simulink model "Simulink_Simulation"  (R2020a)
settings: Solver=ode23tb  StartTime=0.0  StopTime=10.0  RelTol=1e-3  EnableMultiTasking=on
undefined symbols (not defined in the file or in its folder): sigbuilder_block
libraries: powerlib x8
settings Model: Creator=LENOVO  LastModifiedBy=x64
settings DataIOCC: LimitDataPoints=on  SaveFormat=Array  ReturnWorkspaceOutputs=off
settings OptimizationCC: LifeSpan=inf
settings DebuggingCC: SolverPrmCheckMsg=warning  SFUnexpectedBacktrackingDiag=warning  SFNoUnconditionalDefaultTransitionDiag=warning  SFExecutionAtInitializationDiag=none  ArithmeticOperatorsInVariantConditions=warning
settings HardwareCC: ProdBitPerPointer=32  ProdBitPerSizeT=32  ProdBitPerPtrDiffT=32  ProdLargestAtomicFloat=None  ProdIntDivRoundTo=Undefined  ProdEndianess=Unspecified  ProdWordSize=32  ProdHWDeviceType=32-bit Generic
settings ModelReferenceCC: PropagateSignalLabelsOutOfModel=off
settings SFSimCC: SimUseLocalCustomCode=off  CustomCodeUndefinedFunction=UseInterfaceOnly
settings RTWCC: RTWUseLocalCustomCode=off
settings CodeAppCC: StateflowObjectComments=on
settings GRTTargetCC: TargetLangStandard=C89/C90 (ANSI)
settings ConfigComp: CovMetricSettings=dw  CovHtmlReporting=on  CovSaveCumulativeToWorkspaceVar=on  CovSaveSingleToWorkspaceVar=on  CovExternalEMLEnable=off  CovSFcnEnable=off
settings SimscapeCC: SimscapeNormalizeSystem=off

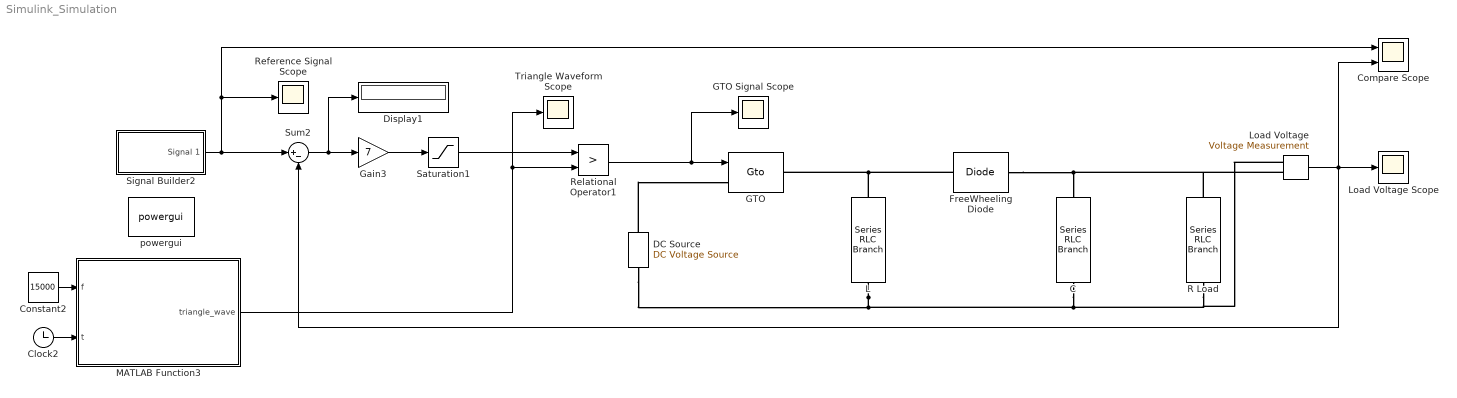
== system Simulink_Simulation ==
  " L" : powerlib/Elements/Series RLC Branch  LConnTagsString=__new0  RConnTagsString=__new0  BranchType=L  Resistance=1  Inductance=3*(1e-4)  SetiL0=off  InitialCurrent=0  Capacitance=1e-6  Setx0=off  InitialVoltage=0  Measurements=None
  " R Load" : powerlib/Elements/Series RLC Branch  LConnTagsString=__new0  RConnTagsString=__new0  BranchType=R  Resistance=100  Inductance=1e-3  SetiL0=off  InitialCurrent=0  Capacitance=1e-6  Setx0=off  InitialVoltage=0  Measurements=None
  C : powerlib/Elements/Series RLC Branch  LConnTagsString=__new0  RConnTagsString=__new0  BranchType=C  Resistance=1  Inductance=1e-3  SetiL0=off  InitialCurrent=0  Capacitance=(1e-6)*250  Setx0=off  InitialVoltage=0  Measurements=None
  Clock2 : Clock
  Compare Scope : Scope  NumInputPorts=2
  Constant2 : Constant  Value=15000
  DC Source : powerlib/Electrical Sources/DC Voltage Source  Amplitude=15  Measurements=None
  Display1 : Display
  FreeWheeling Diode : powerlib/Power Electronics/Diode  Ron=0.01  Lon=0.01  Vf=1  IC=0  UseSnubber=off  Rs=5000  Cs=250e-2  Measurements=off
  GTO : powerlib/Power Electronics/Gto  Ron=0.01  Lon=0.01  Vf=0.8  Tf=10e-6  Tt=20e-7  IC=0  Rs=10000  Cs=inf  Measurements=off
      settings: SourceProductBaseCode=PS
  GTO Signal Scope : Scope
  Gain3 : Gain  Gain=7
  Load Voltage : powerlib/Measurements/Voltage Measurement  PhasorSimulation=off  OutputType=Complex  PSBequivalent=0
  "Load Voltage Scope " : Scope
  MATLAB Function3 : MATLAB Function  TreatAsAtomicUnit=on
  Reference Signal Scope : Scope
  Relational Operator1 : RelationalOperator  Operator=>  OutDataTypeStr=boolean  RndMeth=Nearest
  Saturation1 : Saturate
  Signal Builder2 : Subsystem  Tag=STV Subsys  LoadFcn=sigbuilder_block('load');  StartFcn=sigbuilder_block('start');  StopFcn=sigbuilder_block('stop');  ClipboardFcn=sigbuilder_block('clipboard');  mask(Sigbuilder block){tuvar=[0:10]}
      mask help: Simulink:masks:SigbuilderBlock_MD
      mask init:
      | if ~strcmp(get_param(bdroot(gcbh),'SimulationStatus'),'stopped') tuvar = sigbuilder_block('maskInit'); end
      settings: CopyFcn=sigbuilder_block('copy');  DeleteFcn=sigbuilder_block('delete');  ModelCloseFcn=sigbuilder_block('modelClose');  PreSaveFcn=sigbuilder_block('preSave');  PauseFcn=sigbuilder_block('pause');  ContinueFcn=sigbuilder_block('continue');  NameChangeFcn=sigbuilder_block('namechange');  OpenFcn=sigbuilder_block('open',[0 30 1152 561.6 ]);  CloseFcn=sigbuilder_block('close');
      mask Display: plot(0, 0, 100, 100,[2, 2, 32, 32, 2], [68, 8, 8, 68, 68],[32, 2], [38, 38], [32, 19, 2],[53, 60, 44], [32, 17, 17, 2],[16, 16, 31, 31]);txt = getActiveGroup(gcbh);text(2, 100, txt,'verticalAlignment', 'top');
  Sum2 : Sum  Inputs=|+-
  Triangle Waveform Scope : Scope
  powergui : powerlib/powergui  Priority=1  SimulationMode=Discrete  SampleTime=1e-006  frequency=60  Iterations=50  frequencyindice=0  Pbase=100e6  ErrMax=1e-4  UnitsV=kV  UnitsW=MW  buscounter=0  FunctionMessages=off  echomessages=off  EnableUseOfTLC=off  CurrentSourceSwitches=off  DisableSnubberDevices=off  DisableRonSwitches=off  DisableVfSwitches=off  DisplayEquations=off  AutomaticDiscreteSolvers=off  SolverType=Tustin  Interpol=off  ExternalGateDelay=off  methode=off  Ts=100  x0status=blocks  SPID=off  SwTol=0  HookPort=off  NonlinearTolerance=1e-4  nMaxIteration=100  ContinueOnMaxIteration=off  RestoreLinks=warning  ResistiveCurrentMeasurement=off  Frange=[0:2:500]  Ylog=off  Xlog=on  ShowGrid=off  save=off  variable=ZData  structure=0  ZoomFFT=off  StartTime=0.0  cycles=1  DisplayStyle=1  fundamental=60  FreqAxis=off  MaxFrequency=1000  frequencyindicesteady=1  RmsSteady=1  display=off
  wires:
  Load Voltage/1 -> Compare Scope/2, "Load Voltage Scope "/1, Sum2/2
  Signal Builder2/1(Signal 1) -> Sum2/1, Compare Scope/1, Reference Signal Scope/1
  Sum2/1 -> Display1/1, Gain3/1
  Relational Operator1/1 -> GTO Signal Scope/1, GTO/1
  Saturation1/1 -> Relational Operator1/1
  Constant2/1 -> MATLAB Function3/1(f)
  Clock2/1 -> MATLAB Function3/2(t)
  Gain3/1 -> Saturation1/1
  MATLAB Function3/1(triangle_wave) -> Triangle Waveform Scope/1, Relational Operator1/2
  connections:
  FreeWheeling Diode/LConn1 -- C/LConn1 -- Load Voltage/LConn2 -- " R Load"/LConn1
  " L"/LConn1 -- FreeWheeling Diode/RConn1 -- GTO/RConn1
  " L"/RConn1 -- Load Voltage/LConn1 -- " R Load"/RConn1 -- C/RConn1 -- DC Source/LConn1
  DC Source/RConn1 -- GTO/LConn1

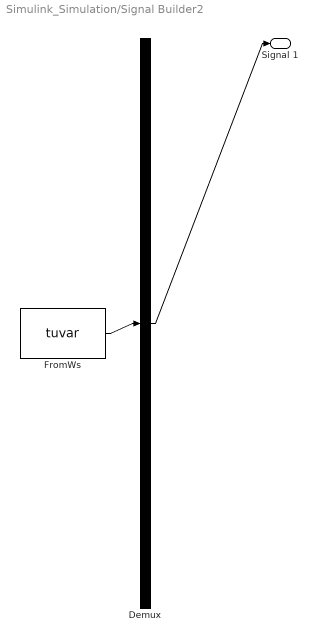
== system Simulink_Simulation/Signal Builder2 ==
  Demux : Demux  Tag=STV Demux  Outputs=1
      settings: DisplayOption=none
  FromWs : FromWorkspace  Tag=STV FromWs  VariableName=tuvar
      SigBuilderData=|
      | common.afterFinalStr = 'Extrapolate'
      | common.sampleTime = 0
      | dataSet.timeRange = [0 10]
      | dataSet.name = 'Group 1'
      | sbobj.Groups.Name = 'Group 1'
      | sbobj.Groups.Signals.Name = 'Signal 1'
      | sbobj.Groups.Signals.XData = [0 1 1 1.5 2.5 3 3 3.5 4 4.5 5 5 5.5 6 6.5 7 7 7.5 7.5 8 8.5 9 9 9.5 10]
      | sbobj.Groups.Signals.YData = [15 15 10 10 10 10 20 20 20 20 20 25 25 25 25 25 5 5 5.05 5 5 5 10 10 10]
  Signal 1 : Outport  Tag=STV Outport
  wires:
  Demux/1 -> Signal 1/1
  FromWs/1 -> Demux/1

== matlab function Simulink_Simulation/MATLAB Function3 ==
  data: f input; triangle_wave output; t input
function triangle_wave = Carrier_Generator(f, t)
%#codegen
% Generates a triangular carrier wave for Buck-Boost Converter PWM
% f: Frequency (Hz), t: Simulation time (clock)

amplitude = 1;
triangle_wave = 0;
multiplier = 1;

half_period = 1/(2*f);             % p
peak_time = half_period/2;         % tepe_zaman

cycle_time = mod(t, 2*half_period);   % t (Current position in full cycle)
local_time = mod(t, half_period);     % zaman (Current position in half cycle)

% Determine polarity based on cycle position
if (cycle_time < half_period)
    multiplier = -1;
else
    multiplier = 1;
end

% Generate Triangle Shape
if (local_time >= peak_time)
    % Falling edge calculation
    triangle_wave = multiplier * ((amplitude/peak_time) * (half_period - local_time));
else
    % Rising edge calculation
    triangle_wave = multiplier * ((amplitude/peak_time) * local_time);
end

return
